simulink model "DDICBF_MO"  (R2022a)
settings: Solver=VariableStepAuto  StartTime=0.0  StopTime=simTime  FixedStep=0.01  RelTol=1e-3
values from neighbouring files (symbols this model uses):
  Kd = 1    [extract_MO.m]
  Kp = 0.2    [extract_MO.m]
  obs = [qO1, qO2, qO3, qO4]    [extract_MO.m]
  qdotstart = [0,0]    [extract_MO.m]
  qg = [2.7, -1.8]    [extract_MO.m]
  qstart = [0,0]    [extract_MO.m]
  r = 0.5    [extract_MO.m]
  threshold_skip = 0.05    [extract_MO.m]
libraries: slctrlblks x1
settings Model: Creator=mirkomizzoni  LastModifiedBy=dennis

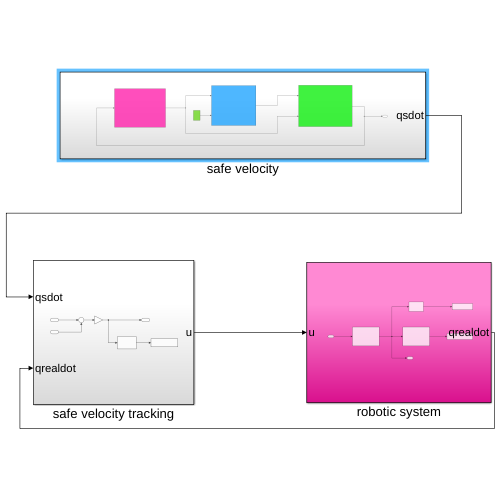
[thumbnail: Simulink's stored preview of the top-level diagram]
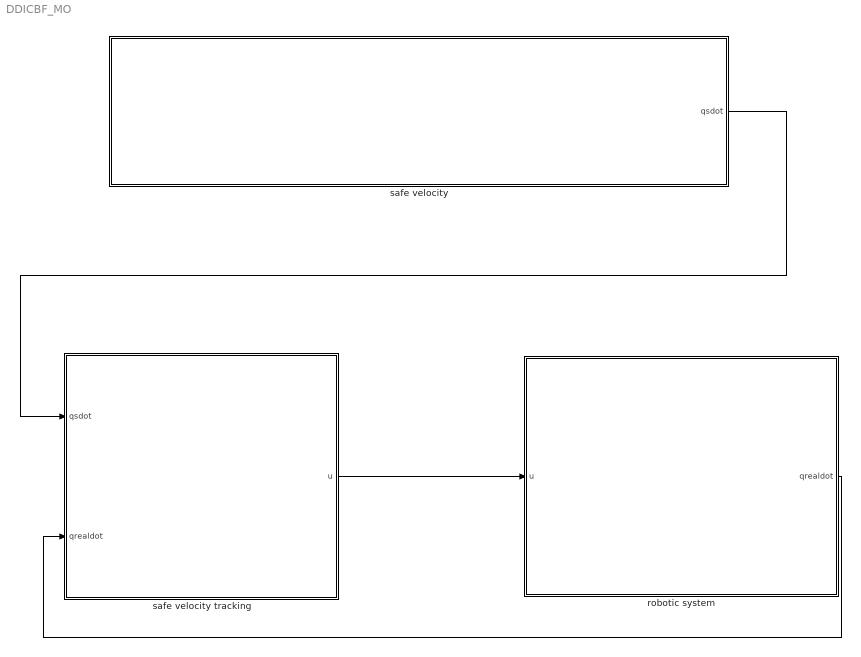
== system DDICBF_MO ==
  robotic system : Subsystem
  safe velocity : Subsystem
  safe velocity tracking : Subsystem
  wires:
  robotic system/1(qrealdot) -> safe velocity tracking/2(qrealdot)
  safe velocity tracking/1(u) -> robotic system/1(u)
  safe velocity/1(qsdot) -> safe velocity tracking/1(qsdot)

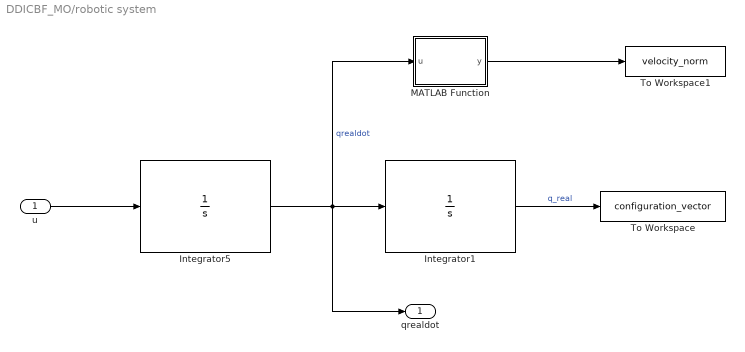
== system DDICBF_MO/robotic system ==
  u : Inport
  Integrator1 : Integrator  InitialCondition=qstart
  Integrator5 : Integrator  InitialCondition=qdotstart
  MATLAB Function : MATLAB Function  TreatAsAtomicUnit=on
  To Workspace : ToWorkspace  VariableName=configuration_vector  SaveFormat=Timeseries  SampleTime=0.01
  To Workspace1 : ToWorkspace  VariableName=velocity_norm  SaveFormat=Timeseries  SampleTime=0.01
  qrealdot : Outport
  wires:
  u/1 -> Integrator5/1
  Integrator5/1 -> qrealdot/1, MATLAB Function/1(u), Integrator1/1  "qrealdot"
  Integrator1/1 -> To Workspace/1  "q_real"
  MATLAB Function/1(y) -> To Workspace1/1

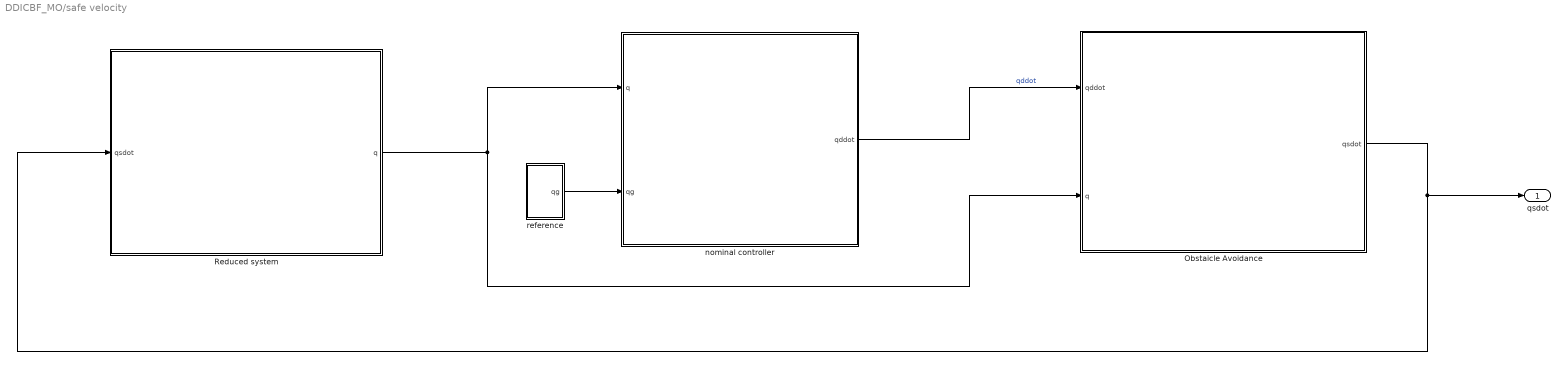
== system DDICBF_MO/safe velocity ==
  Obstaicle Avoidance : Subsystem
  Reduced system : Subsystem
  nominal controller : Subsystem
  reference : Subsystem
  qsdot : Outport
  wires:
  reference/1(qg) -> nominal controller/2(qg)
  Reduced system/1(q) -> Obstaicle Avoidance/2(q), nominal controller/1(q)
  nominal controller/1(qddot) -> Obstaicle Avoidance/1(qddot)  "qddot"
  Obstaicle Avoidance/1(qsdot) -> Reduced system/1(qsdot), qsdot/1

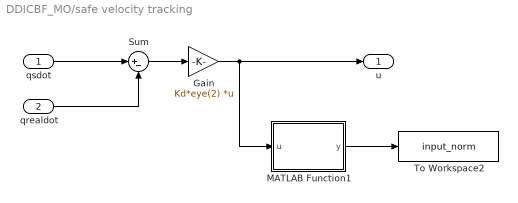
== system DDICBF_MO/safe velocity tracking ==
  qsdot : Inport
  qrealdot : Inport  Port=2
  Gain : Gain  Gain=Kd*eye(2)  Multiplication=Matrix(K*u)
  MATLAB Function1 : MATLAB Function  TreatAsAtomicUnit=on
  Sum : Sum  Inputs=|+-
  To Workspace2 : ToWorkspace  VariableName=input_norm  SaveFormat=Timeseries  SampleTime=0.01
  u : Outport
  wires:
  qrealdot/1 -> Sum/2
  qsdot/1 -> Sum/1
  Sum/1 -> Gain/1
  Gain/1 -> u/1, MATLAB Function1/1(u)
  MATLAB Function1/1(y) -> To Workspace2/1

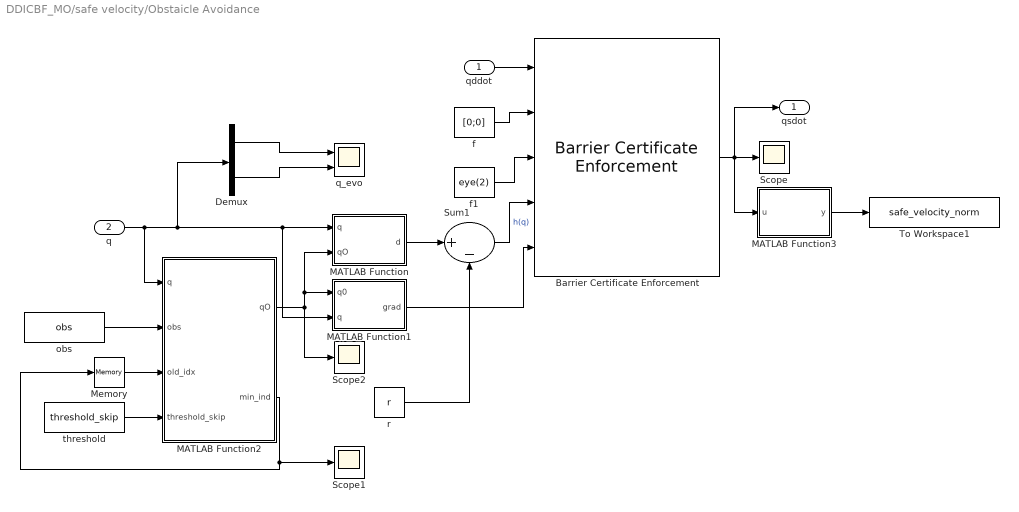
== system DDICBF_MO/safe velocity/Obstaicle Avoidance ==
  qddot : Inport
  q : Inport  Port=2
  Barrier Certificate Enforcement : slctrlblks/Barrier Certificate Enforcement  nx=2  nu=2  nc=1  gamma=alpha  beta=1  external_umax=off  external_umin=off  Ts=0.01  maxiter=200  tol=1e-06  output_exitflag=off
      settings: SourceProductBaseCode=SD
  Demux : Demux  Outputs=2
  MATLAB Function : MATLAB Function  TreatAsAtomicUnit=on
  MATLAB Function1 : MATLAB Function  TreatAsAtomicUnit=on
  MATLAB Function2 : MATLAB Function  TreatAsAtomicUnit=on
  MATLAB Function3 : MATLAB Function  TreatAsAtomicUnit=on
  Memory : Memory  InitialCondition=1
  Scope : Scope
  Scope1 : Scope
  Scope2 : Scope
  Sum1 : Sum  Inputs=|+-
  To Workspace1 : ToWorkspace  VariableName=safe_velocity_norm  SaveFormat=Timeseries  SampleTime=0.01
  f : Constant  Value=[0;0]  VectorParams1D=off
  f1 : Constant  Value=eye(2)  VectorParams1D=off
  obs : Constant  Value=obs  VectorParams1D=off
  q_evo : Scope  NumInputPorts=2
  r : Constant  Value=r
  threshold : Constant  Value=threshold_skip  VectorParams1D=off
  qsdot : Outport
  wires:
  MATLAB Function2/1(qO) -> MATLAB Function/2(qO), MATLAB Function1/1(q0), Scope2/1
  q/1 -> MATLAB Function1/2(q), MATLAB Function/1(q), Demux/1, MATLAB Function2/1(q)
  MATLAB Function2/2(min_ind) -> Memory/1, Scope1/1
  MATLAB Function3/1(y) -> To Workspace1/1
  Sum1/1 -> Barrier Certificate Enforcement/4  "h(q)"
  threshold/1 -> MATLAB Function2/4(threshold_skip)
  f/1 -> Barrier Certificate Enforcement/2
  MATLAB Function1/1(grad) -> Barrier Certificate Enforcement/5
  Demux/1 -> q_evo/1
  qddot/1 -> Barrier Certificate Enforcement/1
  obs/1 -> MATLAB Function2/2(obs)
  Demux/2 -> q_evo/2
  r/1 -> Sum1/2
  f1/1 -> Barrier Certificate Enforcement/3
  Memory/1 -> MATLAB Function2/3(old_idx)
  Barrier Certificate Enforcement/1 -> MATLAB Function3/1(u), Scope/1, qsdot/1
  MATLAB Function/1(d) -> Sum1/1

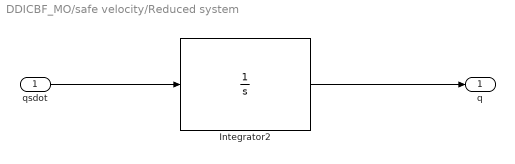
== system DDICBF_MO/safe velocity/Reduced system ==
  qsdot : Inport
  Integrator2 : Integrator  InitialCondition=qstart
  q : Outport
  wires:
  Integrator2/1 -> q/1
  qsdot/1 -> Integrator2/1

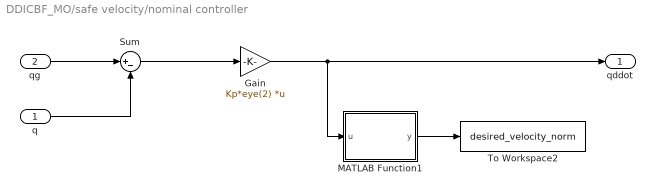
== system DDICBF_MO/safe velocity/nominal controller ==
  q : Inport
  qg : Inport  Port=2
  Gain : Gain  Gain=Kp*eye(2)  Multiplication=Matrix(K*u)
  MATLAB Function1 : MATLAB Function  TreatAsAtomicUnit=on
  Sum : Sum  Inputs=|+-
  To Workspace2 : ToWorkspace  VariableName=desired_velocity_norm  SaveFormat=Timeseries  SampleTime=0.01
  qddot : Outport
  wires:
  MATLAB Function1/1(y) -> To Workspace2/1
  q/1 -> Sum/2
  qg/1 -> Sum/1
  Sum/1 -> Gain/1
  Gain/1 -> qddot/1, MATLAB Function1/1(u)

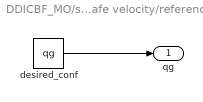
== system DDICBF_MO/safe velocity/reference ==
  desired_conf : Constant  Value=qg
  qg : Outport
  wires:
  desired_conf/1 -> qg/1

== matlab function DDICBF_MO/safe velocity/Obstaicle Avoidance/MATLAB Function1 ==
  data: q0 input; grad output; q input
function grad = gradient(q0,q)
   grad = (q-q0)'/norm(q-q0);
end

== matlab function DDICBF_MO/safe velocity/Obstaicle Avoidance/MATLAB Function ==
  data: q input; qO input; d output
function d = distance(q,qO)
    d = norm(q-qO);
end

== matlab function DDICBF_MO/safe velocity/Obstaicle Avoidance/MATLAB Function2 ==
  data: q input; obs input; qO output; min_ind output; old_idx input; threshold_skip input
function [qO,min_ind] = min_dist(q, obs, old_idx, threshold_skip)
[~,n] = size(obs);
min = norm(q-obs(:,1));
min_ind = 1;
for i=2:n
    t = norm(q-obs(:,i));
    if t<min
        min_ind = i;
        min = t;
    end
end

old_dist = norm(q-obs(:,old_idx));
if abs(old_dist-min) < threshold_skip
    qO = obs(:,old_idx);
    min_ind = old_idx;
    min = old_dist;
else
    qO = obs(:,min_ind);
end

== matlab function DDICBF_MO/robotic system/MATLAB Function ==
  data: u input; y output
function y = norm_func(u)
        
y = norm(u);

== matlab function DDICBF_MO/safe velocity/Obstaicle Avoidance/MATLAB Function3 ==
  data: u input; y output
function y = norm_func(u)
        
y = norm(u);

== matlab function DDICBF_MO/safe velocity tracking/MATLAB Function1 ==
  data: u input; y output
function y = norm_func(u)
        
y = norm(u);

== matlab function DDICBF_MO/safe velocity/nominal controller/MATLAB Function1 ==
  data: u input; y output
function y = norm_func(u)
        
y = norm(u);
